simulink model "pv_dc_converter"  (R2021b)
settings: Solver=VariableStepAuto  StartTime=0.0  StopTime=10.0  RelTol=1e-3
values from neighbouring files (symbols this model uses):
  efficiency_x = efficiency_pv_dcdc(:,1)    [day1.m]    (also in day1_try.m)
  efficiency_y = efficiency_pv_dcdc(:,2)    [day1.m]    (also in day1_try.m)
settings Model: Creator=tinar  LastModifiedBy=tinar

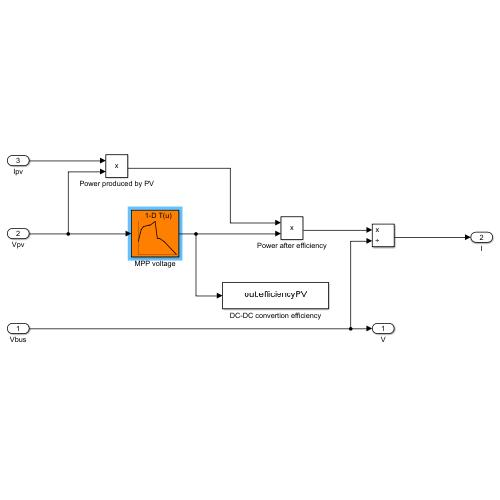
[thumbnail: Simulink's stored preview of the top-level diagram]
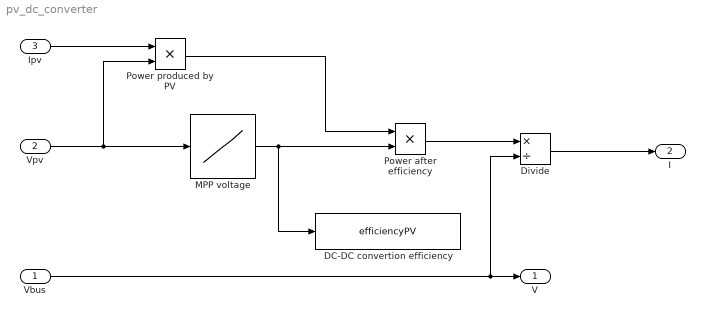
== system pv_dc_converter ==
  Vbus : Inport
  Vpv : Inport  Port=2
  Ipv : Inport  Port=3
  DC-DC convertion efficiency : ToWorkspace  VariableName=efficiencyPV  SaveFormat=Timeseries  SampleTime=-1
  Divide : Product  Inputs=*/
  MPP voltage : Lookup_n-D  NumberOfTableDimensions=1  BreakpointsForDimension1=efficiency_x  Table=efficiency_y  InternalRulePriority=Speed  RndMeth=Simplest  InputSameDT=on
  Power after efficiency : Product
  Power produced by PV : Product
  V : Outport
  I : Outport  Port=2
  wires:
  Ipv/1 -> Power produced by PV/1
  Vpv/1 -> MPP voltage/1, Power produced by PV/2
  Power produced by PV/1 -> Power after efficiency/1
  MPP voltage/1 -> DC-DC convertion efficiency/1, Power after efficiency/2
  Power after efficiency/1 -> Divide/1
  Vbus/1 -> Divide/2, V/1
  Divide/1 -> I/1
